simulink model "closed_loop_8rooms_observer"  (R2022b)
settings: Solver=VariableStepAuto  StartTime=0.0  StopTime=10000  RelTol=1e-3
values from neighbouring files (symbols this model uses):
  A = A .* (1 ./ capacs)    [closed_loop_8rooms.m]    (also in closed_loop_control.m = 100*[-1/capacA * (htAO + htAB + htAC), htAB / capacA,       ; control_time_dependent_A.m = 100*[-1/capacA * (htAO + htAB + htAC), htAB / capacA,       ; open_loop_8rooms.m; open_loop_control.m = 100*[-1/capacA * (htAO + htAB + htAC), htAB / capacA,       )
  B = diag([0 1 0 1 0 1 1 1]) .* (1 ./ capacs)    [closed_loop_8rooms.m]    (also in closed_loop_control.m = [1 / capacA, 0, 0; 0, 1/capacB, 0; 0, 0, 1/capacC]; control_time_dependent_A.m = [1 / capacA, 0, 0; 0, 1/capacB, 0; 0, 0, 1/capacC]; open_loop_8rooms.m; open_loop_control.m = [1 / capacA, 0, 0; 0, 1/capacB, 0; 0, 0, 1/capacC])
  C = diag([0 1 0 1 1 0 0 1])    [closed_loop_8rooms.m]    (also in closed_loop_control.m = [1, 0, 0; 1, 0, 0; 1, 0, 0]; control_time_dependent_A.m = [1, 0, 0; 0, 1, 0; 0, 0, 1]; open_loop_8rooms.m = eye(8); open_loop_control.m = [1, 0, 0; 0, 1, 0; 0, 0, 1])
  D = zeros(8, 8)    [closed_loop_8rooms.m]    (also in closed_loop_control.m = [0, 0, 0; 0, 0, 0; 0, 0, 0]; control_time_dependent_A.m = [0, 0, 0; 0, 0, 0; 0, 0, 0]; open_loop_8rooms.m; open_loop_control.m = [0, 0, 0; 0, 0, 0; 0, 0, 0])
  u_des = -pinv(A\B)*x_des    [closed_loop_8rooms.m]    (also in closed_loop_control.m)
  x0 = [0;0;0;0;0;0;0;0]    [closed_loop_8rooms.m]    (also in closed_loop_control.m = [0;0;0]; control_time_dependent_A.m = [0,0,0]; open_loop_8rooms.m = zeros(8, 1); open_loop_control.m = [0; 0; 0])
  x_des = [20;20;20;20;20;20;20;20]    [closed_loop_8rooms.m]    (also in closed_loop_control.m = [20;20;20]; control_time_dependent_A.m = [20; 20; 20]; open_loop_8rooms.m = [20; 20; 20; 20; 20; 20; 20; 20]; open_loop_control.m = [20; 20; 20])
undefined symbols (not defined in the file or in its folder): K, L
settings Model: Creator=dahliasaba  LastModifiedBy=corlenerhoades
settings OptimizationCC: ReuseModelBlockBuffer=on

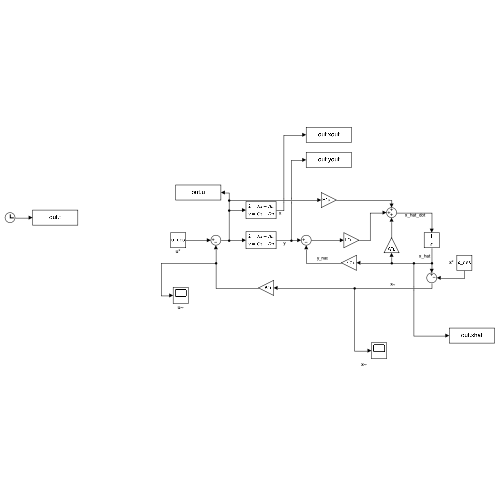
[thumbnail: Simulink's stored preview of the top-level diagram]
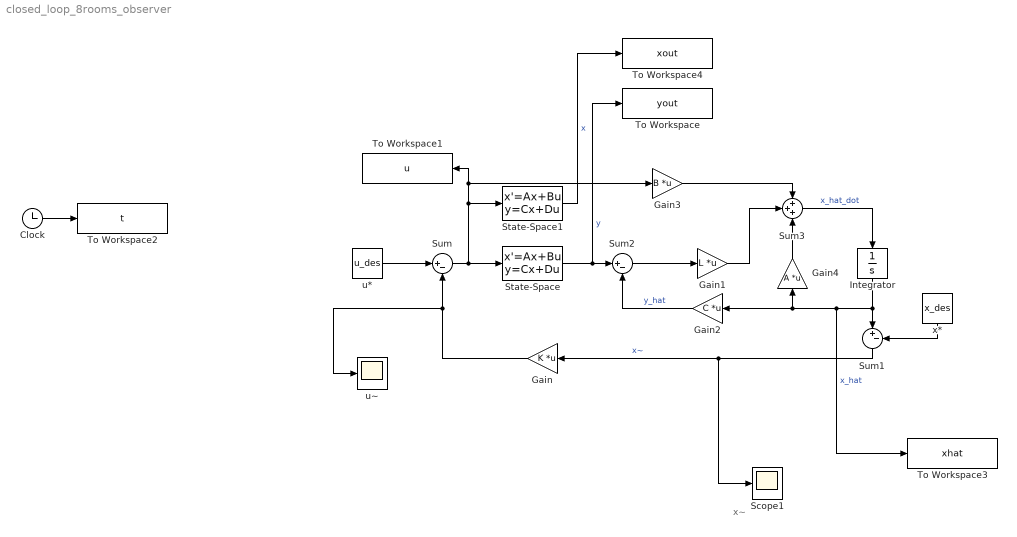
== system closed_loop_8rooms_observer ==
  note: x~
  Clock : Clock
  Gain : Gain  Gain=K  Multiplication=Matrix(K*u)
  Gain1 : Gain  Gain=L  Multiplication=Matrix(K*u)
  Gain2 : Gain  Gain=C  Multiplication=Matrix(K*u)
  Gain3 : Gain  Gain=B  Multiplication=Matrix(K*u)
  Gain4 : Gain  Gain=A  Multiplication=Matrix(K*u)
  Integrator : Integrator
  Scope1 : Scope
  State-Space : StateSpace  A=A  B=B  C=C  D=D  InitialCondition=x0
  State-Space1 : StateSpace  A=A  B=B  C=eye(8)  D=zeros(8,8)  InitialCondition=x0
  Sum : Sum  Inputs=|+-
  Sum1 : Sum  Inputs=|+-
  Sum2 : Sum  Inputs=|+-
  Sum3 : Sum  Inputs=+++
  To Workspace : ToWorkspace  VariableName=yout  SampleTime=-1
  To Workspace1 : ToWorkspace  VariableName=u  SampleTime=-1
  To Workspace2 : ToWorkspace  VariableName=t  SampleTime=-1
  To Workspace3 : ToWorkspace  VariableName=xhat  SampleTime=-1
  To Workspace4 : ToWorkspace  VariableName=xout  SampleTime=-1
  u* : Constant  Value=u_des
  u~ : Scope
  x* : Constant  Value=x_des
  wires:
  u*/1 -> Sum/1
  Sum/1 -> State-Space/1, State-Space1/1, Gain3/1, To Workspace1/1
  Gain/1 -> u~/1, Sum/2
  State-Space/1 -> Sum2/1, To Workspace/1  "y"
  x*/1 -> Sum1/2
  Sum1/1 -> Scope1/1, Gain/1  "x~"
  Clock/1 -> To Workspace2/1
  Integrator/1 -> To Workspace3/1, Gain2/1, Gain4/1, Sum1/1  "x_hat"
  Gain2/1 -> Sum2/2  "y_hat"
  Sum2/1 -> Gain1/1
  Gain1/1 -> Sum3/2
  Gain3/1 -> Sum3/1
  Gain4/1 -> Sum3/3
  Sum3/1 -> Integrator/1  "x_hat_dot"
  State-Space1/1 -> To Workspace4/1  "x"
